simulink library "Driveline_Axle1_None"  (R2025a)
settings: Solver=VariableStepAuto  StartTime=0.0  StopTime=10.0  RelTol=1e-3
libraries: sm_lib x3, Driveshaft_Utilities x1
Description:
  | Component of Simscape Vehicle Templates Library
  | 
  | Copyright 2018-2025 The MathWorks, Inc.
settings Model: Creator=smiller  LastModifiedBy=smiller
settings SolverCC: AlgebraicLoopSolver=TrustRegion
settings DataIOCC: ReturnWorkspaceOutputs=off
settings OptimizationCC: ReuseModelBlockBuffer=off
settings DebuggingCC: UnconnectedInputMsg=warning  UnconnectedOutputMsg=warning  UnconnectedLineMsg=warning  ArithmeticOperatorsInVariantConditions=warning
settings ModelReferenceCC: EnableRefExpFcnMdlSchedulingChecks=on
settings SFSimCC: CustomCodeUndefinedFunction=UseInterfaceOnly
settings RTWCC: GPUComputeCapability=3.5  DLArmComputeVersion=19.05

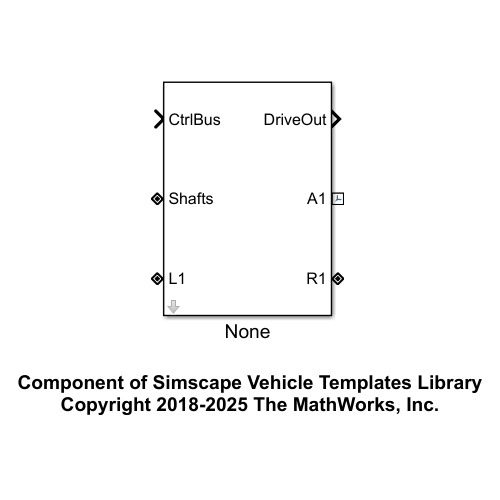
[thumbnail: Simulink's stored preview of the top-level diagram]
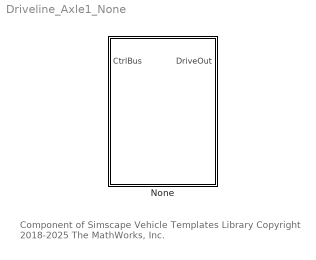
== system Driveline_Axle1_None ==
  note: Component of Simscape Vehicle Templates Library
      | Copyright 2018-2025 The MathWorks, Inc.
  None : Subsystem  Tag=PublishSubsystem  VariantControl=IndepFRDiffFDiffR  mask(Driveline System Placeholder){}
      mask help: Empty subsystem, used as a variant that omits driveline.
      mask Display: disp(' ')

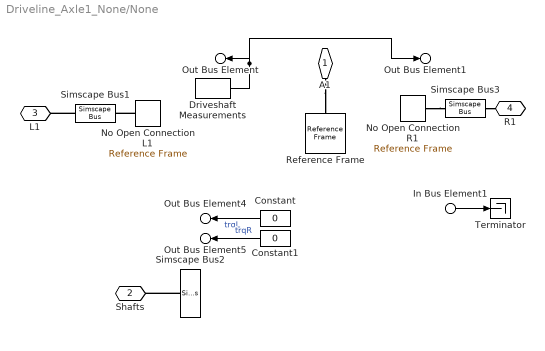
== system Driveline_Axle1_None/None ==
  In Bus Element1 : Inport  PortName=CtrlBus
  Constant : Constant  Value=0
  Constant1 : Constant  Value=0
  Driveshaft Measurements : Driveshaft_Utilities/Driveshaft Measurements  SystemSampleTime=-1  VariantActivationTime=update diagram  EmptyChoice=off  PassThrough=off  PassThroughVariantControl=(default)  EmptyChoiceVariantControl=(default)  AllowFlexibleInterface=on  Latency=0  AutoFrameSizeCalculation=off
  No Open Connection L1 : sm_lib/Frames and Transforms/Reference Frame
  No Open Connection R1 : sm_lib/Frames and Transforms/Reference Frame
  Reference Frame : sm_lib/Frames and Transforms/Reference Frame
  Simscape Bus1 : SimscapeBus  HierarchyStrings=AxleIn
  Simscape Bus2 : SimscapeBus
  Simscape Bus3 : SimscapeBus  HierarchyStrings=AxleIn
  Terminator : Terminator
  A1 : PMIOPort  Side=Right
  Shafts : PMIOPort  Port=2  Side=Left
  L1 : PMIOPort  Port=3  Side=Left
  R1 : PMIOPort  Port=4  Side=Right
  Out Bus Element4 : Outport  VectorParamsAs1DForOutWhenUnconnected=off  PortName=DriveOut  Element=MDriveshaftL1
  Out Bus Element5 : Outport  VectorParamsAs1DForOutWhenUnconnected=off  PortName=DriveOut  Element=MDriveshaftR1
  Out Bus Element : Outport  VectorParamsAs1DForOutWhenUnconnected=off  PortName=DriveOut  Element=anDriveshaftL1
  Out Bus Element1 : Outport  VectorParamsAs1DForOutWhenUnconnected=off  PortName=DriveOut  Element=anDriveshaftR1
  wires:
  Driveshaft Measurements/1 -> Out Bus Element1/1, Out Bus Element/1
  Constant/1 -> Out Bus Element4/1  "trqL"
  Constant1/1 -> Out Bus Element5/1  "trqR"
  In Bus Element1/1 -> Terminator/1
  connections:
  A1/RConn1 -- Reference Frame/RConn1
  Simscape Bus2/RConn1 -- Shafts/RConn1
  Simscape Bus1/RConn1 -- L1/RConn1
  Simscape Bus3/RConn1 -- R1/RConn1
  No Open Connection L1/RConn1 -- Simscape Bus1/LConn1
  No Open Connection R1/RConn1 -- Simscape Bus3/LConn1
